simulink model "Traffic_Light_cs - 原始版本留存"  (R2020a)
settings: Solver=ode5  StartTime=0.0  StopTime=200  FixedStep=1/1000  RelTol=1e-3
PreLoadFcn:
  | mbxruntime.callbacks.PreLoadFcn(bdroot);
PostLoadFcn:
  | mbxruntime.callbacks.PostLoadFcn(bdroot);
InitFcn:
  | mbxruntime.callbacks.InitFcn(bdroot);
StartFcn:
  | mbxruntime.callbacks.StartFcn(bdroot);
StopFcn:
  | mbxruntime.callbacks.StopFcn(bdroot);
model workspace (MAT data in the model file):
  mbox_table : object (value not decoded)
  model_closed = 0
  sim_status = 0
values from neighbouring files (symbols this model uses):
  q_pass = [0 0 0 37.0489514481 49.8894252687 51.0913174965 61.791576133 65.4762304223 75.669686677 80.4628164105 88.6197377629 94.2384891559 ... (437675 elements, 87535x5)]    [Data_ckx.mat]
  q_stop = [0 0 0 15.0544571491 15.7911831418 16.0935138936 18.6666396431 19.4721381181 21.7098800606 22.5642135149 25.0883481215 26.1253405703 ... (437675 elements, 87535x5)]    [Data_ckx.mat]
  s = roadinf.s    [Constraint_T_V.m]    (also in Light_Distinguish_old.m = 75:-0.7:75-84*0.7)
undefined symbols (not defined in the file or in its folder): InitImageOutputDir, mbxruntime, sigbuilder_block, tabledata
libraries: simulink x10, PreScanSimulinkLibrary x8, simulink_extras x4, autolibshared x1, fuzblock x1
(part 3 of 5)

== system Traffic_Light_cs - 原始版本留存/CAR_Main/V2V_Input ==
  TrafficLight_ID_Main : Inport
  Light_Information1 : Inport  Tag=inport/SelfPort  Port=2  PortDimensions=3  SampleTime=1/20  BusOutputAsStruct=on
  Bus Selector1 : BusSelector  OutputSignals=ID_Ahead,LightState_Ahead,TrafficTime_Ahead
  Chart1 : Stateflow chart  TreatAsAtomicUnit=on
  Chart2 : Stateflow chart  Priority=2  TreatAsAtomicUnit=on
  MATLAB Function : MATLAB Function  Priority=1  TreatAsAtomicUnit=on
  Memory : Memory
  Memory1 : Memory
  Memory2 : Memory
  Traffic_State : Outport  VectorParamsAs1DForOutWhenUnconnected=off
  Traffic_Time : Outport  Port=2  VectorParamsAs1DForOutWhenUnconnected=off
  wires:
  Chart1/2(time) -> Traffic_Time/1
  [now_time] -> Chart1/3(now_time)
  MATLAB Function/2(Traffic_now_Time) -> [now_time]  "now_time_Main"
  [State_Next] -> Memory1/1
  [next_time] -> Chart2/3(next_time)
  Chart2/3(localnextID) -> [TrafficID_Next]
  Bus Selector1/2 -> MATLAB Function/3(Light_State_Ahead)  "<LightState_Ahead>"
  TrafficLight_ID_Main/1 -> MATLAB Function/1(Traffic_ID), Chart1/1(TrafficID), Chart2/1(TrafficID)
  [Time_Next] -> Memory2/1
  [now_state] -> Chart1/2(now_state)
  Chart2/1(state) -> [State_Next]
  Bus Selector1/1 -> MATLAB Function/2(TrafficLight_ID_Ahead)  "<ID_Ahead>"
  MATLAB Function/1(Traffic_now_State) -> [now_state]  "now_state_Main"
  MATLAB Function/4(Traffic_next_Time) -> [next_time]  "next_time_Main"
  Bus Selector1/3 -> MATLAB Function/4(Traffic_Time1)  "<TrafficTime_Ahead>"
  Chart1/1(state) -> Traffic_State/1
  Memory2/1 -> MATLAB Function/7(Time_Next)
  Memory/1 -> MATLAB Function/5(TrafficID_Next)
  Memory1/1 -> MATLAB Function/6(State_Next)
  [TrafficID_Next] -> Memory/1
  [next_state] -> Chart2/2(next_state)
  Chart2/2(time) -> [Time_Next]
  MATLAB Function/3(Traffic_next_State) -> [next_state]  "next_state_Main"
  Light_Information1/1 -> Bus Selector1/1

== system Traffic_Light_cs - 原始版本留存/CAR_Main/V2V_Output ==
  Traffic_State : Inport
  Dis_Car2Light_Main : Inport  Port=2
  Light_State_Main : Inport  Port=3
  TrafficLight_ID_Main : Inport  Port=4
  Traffic_Time : Inport  Port=5
  TrafficLight_PhaseTime : Inport  Port=6
  Bus Creator : BusCreator  Inputs=3
  Switch : Switch  Criteria=u2 > Threshold
  Switch1 : Switch  Criteria=u2 > Threshold  Threshold=500
  Traffic_Information : Outport  VectorParamsAs1DForOutWhenUnconnected=off
  "Traffic_Time " : Outport  Port=2  VectorParamsAs1DForOutWhenUnconnected=off
  wires:
  Light_State_Main/1 -> Switch1/3
  Bus Creator/1 -> Traffic_Information/1
  Traffic_State/1 -> Switch1/1
  TrafficLight_PhaseTime/1 -> Switch/3
  Switch1/1 -> Bus Creator/1  "LightState_Main"
  TrafficLight_ID_Main/1 -> Bus Creator/2  "ID_Main"
  Traffic_Time/1 -> Switch/1, Switch/2
  Dis_Car2Light_Main/1 -> Switch1/2
  Switch/1 -> Bus Creator/3, "Traffic_Time "/1  "TrafficTime_Main"

== system Traffic_Light_cs - 原始版本留存/ID_1/VISUCasingLights_Mux ==
  Green [-] : Inport  Tag=inport/Green [-]  SampleTime=1/1000  BusOutputAsStruct=on
  Orange [-] : Inport  Tag=inport/Orange [-]  Port=2  SampleTime=1/1000  BusOutputAsStruct=on
  Red [-] : Inport  Tag=inport/Red [-]  Port=3  SampleTime=1/1000  BusOutputAsStruct=on
  MuxVisuLights : Mux  Inputs=3
  VISUCasingLights_ID_1 : Outport  Tag=outport/VisuCasingLights  SampleTime=1/1000
  wires:
  MuxVisuLights/1 -> VISUCasingLights_ID_1/1
  Green [-]/1 -> MuxVisuLights/1
  Orange [-]/1 -> MuxVisuLights/2
  Red [-]/1 -> MuxVisuLights/3

== system Traffic_Light_cs - 原始版本留存/ID_2/VISUCasingLights_Mux ==
  Green [-] : Inport  Tag=inport/Green [-]  SampleTime=1/1000  BusOutputAsStruct=on
  Orange [-] : Inport  Tag=inport/Orange [-]  Port=2  SampleTime=1/1000  BusOutputAsStruct=on
  Red [-] : Inport  Tag=inport/Red [-]  Port=3  SampleTime=1/1000  BusOutputAsStruct=on
  MuxVisuLights : Mux  Inputs=3
  VISUCasingLights_ID_2 : Outport  Tag=outport/VisuCasingLights  SampleTime=1/1000
  wires:
  MuxVisuLights/1 -> VISUCasingLights_ID_2/1
  Green [-]/1 -> MuxVisuLights/1
  Orange [-]/1 -> MuxVisuLights/2
  Red [-]/1 -> MuxVisuLights/3

== system Traffic_Light_cs - 原始版本留存/ID_3/VISUCasingLights_Mux ==
  Green [-] : Inport  Tag=inport/Green [-]  SampleTime=1/1000  BusOutputAsStruct=on
  Orange [-] : Inport  Tag=inport/Orange [-]  Port=2  SampleTime=1/1000  BusOutputAsStruct=on
  Red [-] : Inport  Tag=inport/Red [-]  Port=3  SampleTime=1/1000  BusOutputAsStruct=on
  MuxVisuLights : Mux  Inputs=3
  VISUCasingLights_ID_3 : Outport  Tag=outport/VisuCasingLights  SampleTime=1/1000
  wires:
  MuxVisuLights/1 -> VISUCasingLights_ID_3/1
  Green [-]/1 -> MuxVisuLights/1
  Orange [-]/1 -> MuxVisuLights/2
  Red [-]/1 -> MuxVisuLights/3

== system Traffic_Light_cs - 原始版本留存/VISUCasingLights_ID_1/Actuator ==
  VISUCasingLights_ID_1 : Inport  Tag=inport/VisuCasingLights  SampleTime=1/1000  BusOutputAsStruct=on
  DemuxVisuLights : Demux  Outputs=3
  LimiterVisuLights : Saturate  UpperLimit=1  LowerLimit=0
  visu_Green [-] : S-Function  FunctionName=sfun_MaterialColorSelector  Parameters=mbxruntime.parameters.convert(UniqueID), mbxruntime.parameters.convert(ColorsObjectQuery), mbxruntime.parameters.convert(Colors),tabledata, TimeStep  SFunctionDeploymentMode=off  EnableBusSupport=off  mask(PreScan Sink Block: VisuTrafficLight){UniqueID=35, ColorsObjectQuery=child:name=ID_1.Casing.LightGreen, Colors=[5   32   25  255    0   64   50  255    0   64   50  255    0    0    0  255; 0   45   34  255    0   45   34  255    0   45   34  255   30  306  240  255], TimeStep=1/1000}
      mask prompts: UniqueID "Parent Unique Identifier"; ColorsObjectQuery "Query for Color Object"; Colors "Matrix of colors"; TimeStep "Simulink time step"
      mask help:
      | The VisuTrafficLight block provides a way to animate traffic lights: switch on and off individual lights.
      |
      | For more information, please click Help.
      mask init:
      | [tabledata] = mbxruntime.parameters.table(UniqueID,ColorsObjectQuery,Colors);
      mask Help: eval('openHelp(731)')
      mask Display: image(imread('TrafficLightCasing.png'))
  visu_Orange [-] : S-Function  FunctionName=sfun_MaterialColorSelector  Parameters=mbxruntime.parameters.convert(UniqueID), mbxruntime.parameters.convert(ColorsObjectQuery), mbxruntime.parameters.convert(Colors),tabledata, TimeStep  SFunctionDeploymentMode=off  EnableBusSupport=off  mask(PreScan Sink Block: VisuTrafficLight){UniqueID=35, ColorsObjectQuery=child:name=ID_1.Casing.LightOrange, Colors=[32   25    5  255   64   48    5  255   64   54    5  255    0    0    0  255; 45   34    0  255   45   34    0  255   45   34    0  255  306  229    5  255], TimeStep=1/1000}
      mask prompts: UniqueID "Parent Unique Identifier"; ColorsObjectQuery "Query for Color Object"; Colors "Matrix of colors"; TimeStep "Simulink time step"
      mask help:
      | The VisuTrafficLight block provides a way to animate traffic lights: switch on and off individual lights.
      |
      | For more information, please click Help.
      mask init:
      | [tabledata] = mbxruntime.parameters.table(UniqueID,ColorsObjectQuery,Colors);
      mask Help: eval('openHelp(731)')
      mask Display: image(imread('TrafficLightCasing.png'))
  visu_Red [-] : S-Function  FunctionName=sfun_MaterialColorSelector  Parameters=mbxruntime.parameters.convert(UniqueID), mbxruntime.parameters.convert(ColorsObjectQuery), mbxruntime.parameters.convert(Colors),tabledata, TimeStep  SFunctionDeploymentMode=off  EnableBusSupport=off  mask(PreScan Sink Block: VisuTrafficLight){UniqueID=35, ColorsObjectQuery=child:name=ID_1.Casing.LightRed, Colors=[32    5    5  255   64    5    5  255   64    5    5  255    0    0    0  255; 45    0    0  255   45    0    0  255   45    0    0  255  306   30   30  255], TimeStep=1/1000}
      mask prompts: UniqueID "Parent Unique Identifier"; ColorsObjectQuery "Query for Color Object"; Colors "Matrix of colors"; TimeStep "Simulink time step"
      mask help:
      | The VisuTrafficLight block provides a way to animate traffic lights: switch on and off individual lights.
      |
      | For more information, please click Help.
      mask init:
      | [tabledata] = mbxruntime.parameters.table(UniqueID,ColorsObjectQuery,Colors);
      mask Help: eval('openHelp(731)')
      mask Display: image(imread('TrafficLightCasing.png'))
  wires:
  VISUCasingLights_ID_1/1 -> LimiterVisuLights/1
  LimiterVisuLights/1 -> DemuxVisuLights/1
  DemuxVisuLights/1 -> visu_Green [-]/1
  DemuxVisuLights/2 -> visu_Orange [-]/1
  DemuxVisuLights/3 -> visu_Red [-]/1

== system Traffic_Light_cs - 原始版本留存/VISUCasingLights_ID_2/Actuator ==
  VISUCasingLights_ID_2 : Inport  Tag=inport/VisuCasingLights  SampleTime=1/1000  BusOutputAsStruct=on
  DemuxVisuLights : Demux  Outputs=3
  LimiterVisuLights : Saturate  UpperLimit=1  LowerLimit=0
  visu_Green [-] : S-Function  FunctionName=sfun_MaterialColorSelector  Parameters=mbxruntime.parameters.convert(UniqueID), mbxruntime.parameters.convert(ColorsObjectQuery), mbxruntime.parameters.convert(Colors),tabledata, TimeStep  SFunctionDeploymentMode=off  EnableBusSupport=off  mask(PreScan Sink Block: VisuTrafficLight){UniqueID=525, ColorsObjectQuery=child:name=ID_2.Casing.LightGreen, Colors=[5   32   25  255    0   64   50  255    0   64   50  255    0    0    0  255; 0   45   34  255    0   45   34  255    0   45   34  255   30  306  240  255], TimeStep=1/1000}
      mask prompts: UniqueID "Parent Unique Identifier"; ColorsObjectQuery "Query for Color Object"; Colors "Matrix of colors"; TimeStep "Simulink time step"
      mask help:
      | The VisuTrafficLight block provides a way to animate traffic lights: switch on and off individual lights.
      |
      | For more information, please click Help.
      mask init:
      | [tabledata] = mbxruntime.parameters.table(UniqueID,ColorsObjectQuery,Colors);
      mask Help: eval('openHelp(731)')
      mask Display: image(imread('TrafficLightCasing.png'))
  visu_Orange [-] : S-Function  FunctionName=sfun_MaterialColorSelector  Parameters=mbxruntime.parameters.convert(UniqueID), mbxruntime.parameters.convert(ColorsObjectQuery), mbxruntime.parameters.convert(Colors),tabledata, TimeStep  SFunctionDeploymentMode=off  EnableBusSupport=off  mask(PreScan Sink Block: VisuTrafficLight){UniqueID=525, ColorsObjectQuery=child:name=ID_2.Casing.LightOrange, Colors=[32   25    5  255   64   48    5  255   64   54    5  255    0    0    0  255; 45   34    0  255   45   34    0  255   45   34    0  255  306  229    5  255], TimeStep=1/1000}
      mask prompts: UniqueID "Parent Unique Identifier"; ColorsObjectQuery "Query for Color Object"; Colors "Matrix of colors"; TimeStep "Simulink time step"
      mask help:
      | The VisuTrafficLight block provides a way to animate traffic lights: switch on and off individual lights.
      |
      | For more information, please click Help.
      mask init:
      | [tabledata] = mbxruntime.parameters.table(UniqueID,ColorsObjectQuery,Colors);
      mask Help: eval('openHelp(731)')
      mask Display: image(imread('TrafficLightCasing.png'))
  visu_Red [-] : S-Function  FunctionName=sfun_MaterialColorSelector  Parameters=mbxruntime.parameters.convert(UniqueID), mbxruntime.parameters.convert(ColorsObjectQuery), mbxruntime.parameters.convert(Colors),tabledata, TimeStep  SFunctionDeploymentMode=off  EnableBusSupport=off  mask(PreScan Sink Block: VisuTrafficLight){UniqueID=525, ColorsObjectQuery=child:name=ID_2.Casing.LightRed, Colors=[32    5    5  255   64    5    5  255   64    5    5  255    0    0    0  255; 45    0    0  255   45    0    0  255   45    0    0  255  306   30   30  255], TimeStep=1/1000}
      mask prompts: UniqueID "Parent Unique Identifier"; ColorsObjectQuery "Query for Color Object"; Colors "Matrix of colors"; TimeStep "Simulink time step"
      mask help:
      | The VisuTrafficLight block provides a way to animate traffic lights: switch on and off individual lights.
      |
      | For more information, please click Help.
      mask init:
      | [tabledata] = mbxruntime.parameters.table(UniqueID,ColorsObjectQuery,Colors);
      mask Help: eval('openHelp(731)')
      mask Display: image(imread('TrafficLightCasing.png'))
  wires:
  VISUCasingLights_ID_2/1 -> LimiterVisuLights/1
  LimiterVisuLights/1 -> DemuxVisuLights/1
  DemuxVisuLights/1 -> visu_Green [-]/1
  DemuxVisuLights/2 -> visu_Orange [-]/1
  DemuxVisuLights/3 -> visu_Red [-]/1

== system Traffic_Light_cs - 原始版本留存/VISUCasingLights_ID_3/Actuator ==
  VISUCasingLights_ID_3 : Inport  Tag=inport/VisuCasingLights  SampleTime=1/1000  BusOutputAsStruct=on
  DemuxVisuLights : Demux  Outputs=3
  LimiterVisuLights : Saturate  UpperLimit=1  LowerLimit=0
  visu_Green [-] : S-Function  FunctionName=sfun_MaterialColorSelector  Parameters=mbxruntime.parameters.convert(UniqueID), mbxruntime.parameters.convert(ColorsObjectQuery), mbxruntime.parameters.convert(Colors),tabledata, TimeStep  SFunctionDeploymentMode=off  EnableBusSupport=off  mask(PreScan Sink Block: VisuTrafficLight){UniqueID=526, ColorsObjectQuery=child:name=ID_3.Casing.LightGreen, Colors=[5   32   25  255    0   64   50  255    0   64   50  255    0    0    0  255; 0   45   34  255    0   45   34  255    0   45   34  255   30  306  240  255], TimeStep=1/1000}
      mask prompts: UniqueID "Parent Unique Identifier"; ColorsObjectQuery "Query for Color Object"; Colors "Matrix of colors"; TimeStep "Simulink time step"
      mask help:
      | The VisuTrafficLight block provides a way to animate traffic lights: switch on and off individual lights.
      |
      | For more information, please click Help.
      mask init:
      | [tabledata] = mbxruntime.parameters.table(UniqueID,ColorsObjectQuery,Colors);
      mask Help: eval('openHelp(731)')
      mask Display: image(imread('TrafficLightCasing.png'))
  visu_Orange [-] : S-Function  FunctionName=sfun_MaterialColorSelector  Parameters=mbxruntime.parameters.convert(UniqueID), mbxruntime.parameters.convert(ColorsObjectQuery), mbxruntime.parameters.convert(Colors),tabledata, TimeStep  SFunctionDeploymentMode=off  EnableBusSupport=off  mask(PreScan Sink Block: VisuTrafficLight){UniqueID=526, ColorsObjectQuery=child:name=ID_3.Casing.LightOrange, Colors=[32   25    5  255   64   48    5  255   64   54    5  255    0    0    0  255; 45   34    0  255   45   34    0  255   45   34    0  255  306  229    5  255], TimeStep=1/1000}
      mask prompts: UniqueID "Parent Unique Identifier"; ColorsObjectQuery "Query for Color Object"; Colors "Matrix of colors"; TimeStep "Simulink time step"
      mask help:
      | The VisuTrafficLight block provides a way to animate traffic lights: switch on and off individual lights.
      |
      | For more information, please click Help.
      mask init:
      | [tabledata] = mbxruntime.parameters.table(UniqueID,ColorsObjectQuery,Colors);
      mask Help: eval('openHelp(731)')
      mask Display: image(imread('TrafficLightCasing.png'))
  visu_Red [-] : S-Function  FunctionName=sfun_MaterialColorSelector  Parameters=mbxruntime.parameters.convert(UniqueID), mbxruntime.parameters.convert(ColorsObjectQuery), mbxruntime.parameters.convert(Colors),tabledata, TimeStep  SFunctionDeploymentMode=off  EnableBusSupport=off  mask(PreScan Sink Block: VisuTrafficLight){UniqueID=526, ColorsObjectQuery=child:name=ID_3.Casing.LightRed, Colors=[32    5    5  255   64    5    5  255   64    5    5  255    0    0    0  255; 45    0    0  255   45    0    0  255   45    0    0  255  306   30   30  255], TimeStep=1/1000}
      mask prompts: UniqueID "Parent Unique Identifier"; ColorsObjectQuery "Query for Color Object"; Colors "Matrix of colors"; TimeStep "Simulink time step"
      mask help:
      | The VisuTrafficLight block provides a way to animate traffic lights: switch on and off individual lights.
      |
      | For more information, please click Help.
      mask init:
      | [tabledata] = mbxruntime.parameters.table(UniqueID,ColorsObjectQuery,Colors);
      mask Help: eval('openHelp(731)')
      mask Display: image(imread('TrafficLightCasing.png'))
  wires:
  VISUCasingLights_ID_3/1 -> LimiterVisuLights/1
  LimiterVisuLights/1 -> DemuxVisuLights/1
  DemuxVisuLights/1 -> visu_Green [-]/1
  DemuxVisuLights/2 -> visu_Orange [-]/1
  DemuxVisuLights/3 -> visu_Red [-]/1

== system Traffic_Light_cs - 原始版本留存/CAR_Ahead/Decision/Function-Call Subsystem ==
  Dis : Inport
  "CameraSensor " : Inport  Port=2
  Traffic_State : Inport  Port=3
  Traffic_Time : Inport  Port=4
  V_now : Inport  Port=5
  function : TriggerPort  TriggerType=function-call  VariantControl=Variant
  Chart : Stateflow chart  TreatAsAtomicUnit=on
  Subsystem : Subsystem
  Switch : Switch  Criteria=u2 > Threshold
  Terminator : Terminator
  Terminator1 : Terminator
  Light_State_Ahead : Outport  VectorParamsAs1DForOutWhenUnconnected=off
  wires:
  V_now/1 -> Terminator1/1
  Traffic_Time/1 -> Terminator/1, [TrafficTime]
  Subsystem/1(Light_State_Ahead) -> Switch/3
  Switch/1 -> Light_State_Ahead/1, [LightState]
  Chart/1(Camera_Call()) -> Subsystem/Trigger
  Traffic_State/1 -> Chart/1(Traffic_State), Switch/1, Switch/2
  "CameraSensor "/1 -> Subsystem/2("CameraSensor ")
  Dis/1 -> Subsystem/1(Dis), [Distance]

== system Traffic_Light_cs - 原始版本留存/CAR_Ahead/SELF_Demux/compas converter ==
  rotz [rad] : Inport
  cart2compas : Subsystem
  rad2deg : Gain  Gain=180/pi
  heading [deg] : Outport
  wires:
  rad2deg/1 -> cart2compas/1(Angle [deg])
  rotz [rad]/1 -> rad2deg/1
  cart2compas/1(heading [deg]) -> heading [deg]/1

== system Traffic_Light_cs - 原始版本留存/CAR_Ahead/Subsystem/Signal Builder ==
  Demux : Demux  Tag=STV Demux  Outputs=6
      settings: DisplayOption=none
  FromWs : FromWorkspace  Tag=STV FromWs  VariableName=tuvar
      SigBuilderData=|
      | common.afterFinalStr = 'Extrapolate'
      | common.sampleTime = 0
      | dataSet.timeRange = [0 200]
      | dataSet.name = 'Traffic Light GPS Information'
      | sbobj.Groups.Name = 'Traffic Light GPS Information'
      | sbobj.Groups.Signals(1).Name = 'ID==1,X'
      | sbobj.Groups.Signals(1).XData = [0 200]
      | sbobj.Groups.Signals(1).YData = [-610.5 -610.5]
      | sbobj.Groups.Signals(2).Name = 'ID==1,Y'
      | sbobj.Groups.Signals(2).XData = [0 200]
      | sbobj.Groups.Signals(2).YData = [362.27 362.27]
      | sbobj.Groups.Signals(3).Name = 'ID==2,X'
      | sbobj.Groups.Signals(3).XData = [0 200]
      | sbobj.Groups.Signals(3).YData = [-639.42 -639.42]
      | sbobj.Groups.Signals(4).Name = 'ID==2,Y'
      | sbobj.Groups.Signals(4).XData = [0 200]
      | sbobj.Groups.Signals(4).YData = [295.94 295.94]
      | sbobj.Groups.Signals(5).Name = 'ID==3,X'
      | sbobj.Groups.Signals(5).XData = [0 200]
      | sbobj.Groups.Signals(5).YData = [-718.98 -718.98]
      | sbobj.Groups.Signals(6).Name = 'ID==3,Y'
      | sbobj.Groups.Signals(6).XData = [0 200]
      | sbobj.Groups.Signals(6).YData = [201.74 201.74]
      | sbobj.Groups.TimeRange = [0 200]
  ID==1,X : Outport  Tag=STV Outport
  ID==1,Y : Outport  Tag=STV Outport  Port=2  VectorParamsAs1DForOutWhenUnconnected=off
  ID==2,X : Outport  Tag=STV Outport  Port=3  VectorParamsAs1DForOutWhenUnconnected=off
  ID==2,Y : Outport  Tag=STV Outport  Port=4  VectorParamsAs1DForOutWhenUnconnected=off
  ID==3,X : Outport  Tag=STV Outport  Port=5  VectorParamsAs1DForOutWhenUnconnected=off
  ID==3,Y : Outport  Tag=STV Outport  Port=6  VectorParamsAs1DForOutWhenUnconnected=off
  wires:
  Demux/6 -> ID==3,Y/1
  Demux/5 -> ID==3,X/1
  Demux/4 -> ID==2,Y/1
  Demux/3 -> ID==2,X/1
  Demux/2 -> ID==1,Y/1
  Demux/1 -> ID==1,X/1
  FromWs/1 -> Demux/1

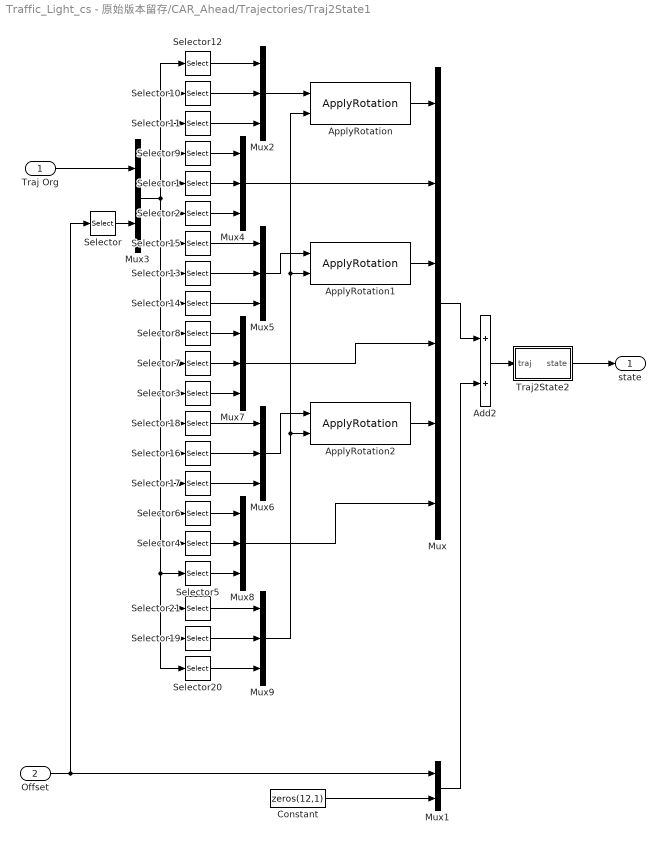
== system Traffic_Light_cs - 原始版本留存/CAR_Ahead/Trajectories/Traj2State1 ==
  Traj Org : Inport
  Offset : Inport  Port=2
  Add2 : Sum
  ApplyRotation : PreScanSimulinkLibrary/ApplyRotation  SystemSampleTime=-1  Latency=0  AutoFrameSizeCalculation=off
  ApplyRotation1 : PreScanSimulinkLibrary/ApplyRotation  SystemSampleTime=-1  Latency=0  AutoFrameSizeCalculation=off
  ApplyRotation2 : PreScanSimulinkLibrary/ApplyRotation  SystemSampleTime=-1  Latency=0  AutoFrameSizeCalculation=off
  Constant : Constant  Value=zeros(12,1)
  Mux : Mux  Inputs=6
  Mux1 : Mux  Inputs=2
  Mux{2,4..9} (7 alike) : Mux  Inputs=3
  Mux3 : Mux  Inputs=2
  Selector : Selector  InputPortWidth=6  IndexOptions=Index vector (dialog)  Indices=[4 5 6]  OutputSizes=1
  Selector1 : Selector  InputPortWidth=21  IndexOptions=Index vector (dialog)  Indices=[5]  OutputSizes=1
  Selector10 : Selector  InputPortWidth=21  IndexOptions=Index vector (dialog)  Indices=[2]  OutputSizes=1
  Selector11 : Selector  InputPortWidth=21  IndexOptions=Index vector (dialog)  Indices=[3]  OutputSizes=1
  Selector12 : Selector  InputPortWidth=21  IndexOptions=Index vector (dialog)  Indices=[1]  OutputSizes=1
  Selector13 : Selector  InputPortWidth=21  IndexOptions=Index vector (dialog)  Indices=[8]  OutputSizes=1
  Selector14 : Selector  InputPortWidth=21  IndexOptions=Index vector (dialog)  Indices=[9]  OutputSizes=1
  Selector15 : Selector  InputPortWidth=21  IndexOptions=Index vector (dialog)  Indices=[7]  OutputSizes=1
  Selector16 : Selector  InputPortWidth=21  IndexOptions=Index vector (dialog)  Indices=[14]  OutputSizes=1
  Selector17 : Selector  InputPortWidth=21  IndexOptions=Index vector (dialog)  Indices=[15]  OutputSizes=1
  Selector18 : Selector  InputPortWidth=21  IndexOptions=Index vector (dialog)  Indices=[13]  OutputSizes=1
  Selector19 : Selector  InputPortWidth=21  IndexOptions=Index vector (dialog)  Indices=[20]  OutputSizes=1
  Selector2 : Selector  InputPortWidth=21  IndexOptions=Index vector (dialog)  Indices=[6]  OutputSizes=1
  Selector20 : Selector  InputPortWidth=21  IndexOptions=Index vector (dialog)  Indices=[21]  OutputSizes=1
  Selector21 : Selector  InputPortWidth=21  IndexOptions=Index vector (dialog)  Indices=[19]  OutputSizes=1
  Selector3 : Selector  InputPortWidth=21  IndexOptions=Index vector (dialog)  Indices=[12]  OutputSizes=1
  Selector4 : Selector  InputPortWidth=21  IndexOptions=Index vector (dialog)  Indices=[17]  OutputSizes=1
  Selector5 : Selector  InputPortWidth=21  IndexOptions=Index vector (dialog)  Indices=[18]  OutputSizes=1
  Selector6 : Selector  InputPortWidth=21  IndexOptions=Index vector (dialog)  Indices=[16]  OutputSizes=1
  Selector7 : Selector  InputPortWidth=21  IndexOptions=Index vector (dialog)  Indices=[11]  OutputSizes=1
  Selector8 : Selector  InputPortWidth=21  IndexOptions=Index vector (dialog)  Indices=[10]  OutputSizes=1
  Selector9 : Selector  InputPortWidth=21  IndexOptions=Index vector (dialog)  Indices=[4]  OutputSizes=1
  Traj2State2 : Subsystem
  state : Outport
  wires:
  Mux9/1 -> ApplyRotation2/2, ApplyRotation1/2, ApplyRotation/2
  Selector20/1 -> Mux9/3
  Selector19/1 -> Mux9/2
  Selector21/1 -> Mux9/1
  Selector5/1 -> Mux8/3
  Selector4/1 -> Mux8/2
  Selector6/1 -> Mux8/1
  Mux8/1 -> Mux/6
  Mux6/1 -> ApplyRotation2/1
  Mux7/1 -> Mux/4
  ApplyRotation2/1 -> Mux/5
  Selector3/1 -> Mux7/3
  Selector7/1 -> Mux7/2
  Selector8/1 -> Mux7/1
  Mux4/1 -> Mux/2
  Mux5/1 -> ApplyRotation1/1
  ApplyRotation1/1 -> Mux/3
  Mux2/1 -> ApplyRotation/1
  ApplyRotation/1 -> Mux/1
  Selector2/1 -> Mux4/3
  Selector1/1 -> Mux4/2
  Selector9/1 -> Mux4/1
  Selector17/1 -> Mux6/3
  Selector16/1 -> Mux6/2
  Selector18/1 -> Mux6/1
  Selector14/1 -> Mux5/3
  Selector13/1 -> Mux5/2
  Selector15/1 -> Mux5/1
  Selector11/1 -> Mux2/3
  Selector10/1 -> Mux2/2
  Selector12/1 -> Mux2/1
  Mux3/1 -> Selector8/1, Selector7/1, Selector3/1, Selector18/1, Selector16/1, Selector17/1, Selector6/1, Selector20/1, Selector19/1, Selector21/1, Selector5/1, Selector4/1, Selector14/1, Selector13/1, Selector15/1, Selector2/1, Selector1/1, Selector9/1, Selector12/1, Selector10/1, Selector11/1
  Mux1/1 -> Add2/2
  Constant/1 -> Mux1/2
  Add2/1 -> Traj2State2/1(traj)
  Selector/1 -> Mux3/2
  Traj Org/1 -> Mux3/1
  Offset/1 -> Mux1/1, Selector/1
  Mux/1 -> Add2/1
  Traj2State2/1(state) -> state/1

== system Traffic_Light_cs - 原始版本留存/CAR_Ahead/Trajectories/TrajCoGOffset ==
  State In : Inport
  Add : Sum  Inputs=+-+
  Add1 : Sum
  ApplyRotation : PreScanSimulinkLibrary/ApplyRotation  SystemSampleTime=-1  Latency=0  AutoFrameSizeCalculation=off
  ApplyRotation1 : PreScanSimulinkLibrary/ApplyRotation  SystemSampleTime=-1  Latency=0  AutoFrameSizeCalculation=off
  CoG Offset : Constant  Value=[0 0 CoGOffsetZ]
  Degrees to Radians : simulink_extras/Transformations/Degrees to Radians
  Demux1 : Demux  Outputs=[3 3 3]
  Mux : Mux  Inputs=[3 3 3]
  Orientation : Constant  Value=[InitRoll InitPitch 0]
  State Out : Outport
  wires:
  State In/1 -> Demux1/1
  Demux1/1 -> Add/1
  Add/1 -> Mux/1
  Demux1/3 -> Mux/3, Add1/2
  Mux/1 -> State Out/1
  Demux1/2 -> Mux/2
  Orientation/1 -> Degrees to Radians/1
  ApplyRotation/1 -> Add/3
  ApplyRotation1/1 -> Add/2
  Add1/1 -> ApplyRotation/2
  CoG Offset/1 -> ApplyRotation1/1, ApplyRotation/1
  Degrees to Radians/1 -> Add1/1, ApplyRotation1/2

== system Traffic_Light_cs - 原始版本留存/CAR_Ahead/Trajectories/Trajectory_1 ==
  From Workspace : FromWorkspace  VariableName=trajectory  SampleTime=TimeStep  ZeroCross=off  OutputAfterFinalValue=Holding final value
  From Workspace1 : FromWorkspace  VariableName=trajectory  SampleTime=TimeStep  ZeroCross=off  OutputAfterFinalValue=Setting to zero
  Mux : Mux  Inputs=2
  Selector1 : Selector  InputPortWidth=24  IndexOptions=Index vector (dialog)  Indices=[7:18]  OutputSizes=1
  Selector9 : Selector  InputPortWidth=24  IndexOptions=Index vector (dialog)  Indices=[1:6]  OutputSizes=1
  trajectory : Outport
  wires:
  From Workspace/1 -> Selector9/1
  From Workspace1/1 -> Selector1/1
  Mux/1 -> trajectory/1
  Selector9/1 -> Mux/1
  Selector1/1 -> Mux/2

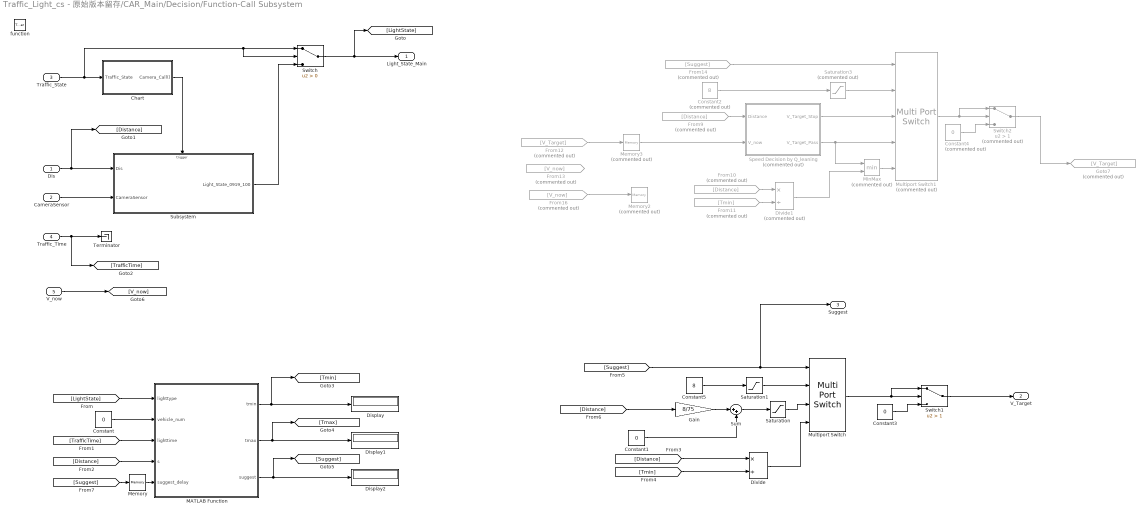
== system Traffic_Light_cs - 原始版本留存/CAR_Main/Decision/Function-Call Subsystem ==
  Dis : Inport
  "CameraSensor " : Inport  Port=2
  Traffic_State : Inport  Port=3
  Traffic_Time : Inport  Port=4
  V_now : Inport  Port=5
  function : TriggerPort  TriggerType=function-call  VariantControl=Variant
  Chart : Stateflow chart  TreatAsAtomicUnit=on
  Constant : Constant  Value=0
  Constant1 : Constant  Value=0
  Constant2 : Constant  Commented=on  Value=8
  Constant3 : Constant  Value=0
  Constant4 : Constant  Commented=on  Value=0
  Constant5 : Constant  Value=8
  Display : Display
  Display1 : Display
  Display2 : Display
  Divide : Product  Inputs=*/
  Divide1 : Product  Commented=on  Inputs=*/
  From10 : From  Commented=on  GotoTag=Distance
  From11 : From  Commented=on  GotoTag=Tmin
  From12 : From  Commented=on  GotoTag=V_Target
  From13 : From  Commented=on  GotoTag=V_now
  From14 : From  Commented=on  GotoTag=Suggest
  From16 : From  Commented=on  GotoTag=V_now
  From9 : From  Commented=on  GotoTag=Distance
  Gain : Gain  Gain=8/75
  Goto7 : Goto  Commented=on  GotoTag=V_Target
  MATLAB Function : MATLAB Function  TreatAsAtomicUnit=on
  Memory : Memory  InheritSampleTime=on
  Memory2 : Memory  Commented=on  InitialCondition=6  InheritSampleTime=on
  Memory3 : Memory  Commented=on  InitialCondition=3  InheritSampleTime=on
  MinMax : MinMax  Commented=on  Inputs=2
  Multiport Switch : MultiPortSwitch  DataPortOrder=Specify indices  DataPortIndices={-1,4,3}  DiagnosticForDefault=None
  Multiport Switch1 : MultiPortSwitch  Commented=on  DataPortOrder=Specify indices  DataPortIndices={-1,4,1,3}  DiagnosticForDefault=None
  Saturation : Saturate  UpperLimit=10  LowerLimit=0
  Saturation1 : Saturate  UpperLimit=20  LowerLimit=5
  Saturation3 : Saturate  Commented=on  UpperLimit=20  LowerLimit=0
  Speed Decision by Q_leaning : Subsystem  Commented=on
  Subsystem : Subsystem
  Sum : Sum  Inputs=|++
  Switch : Switch  Criteria=u2 > Threshold
  Switch1 : Switch  Criteria=u2 > Threshold  Threshold=1
  Switch2 : Switch  Commented=on  Criteria=u2 > Threshold  Threshold=1
  Terminator : Terminator
  Light_State_Main : Outport  VectorParamsAs1DForOutWhenUnconnected=off
  V_Target : Outport  Port=2  VectorParamsAs1DForOutWhenUnconnected=off
  "Suggest " : Outport  Port=3  VectorParamsAs1DForOutWhenUnconnected=off
  wires:
  Constant5/1 -> Saturation1/1
  Switch1/1 -> V_Target/1
  Constant2/1 -> Saturation3/1
  Memory3/1 -> Speed Decision by Q_leaning/2(V_now)
  From12/1 -> Memory3/1
  From16/1 -> Memory2/1
  MinMax/1 -> Multiport Switch1/5
  Divide1/1 -> MinMax/2
  Speed Decision by Q_leaning/2(V_Target_Pass) -> Multiport Switch1/4, MinMax/1
  From10/1 -> Divide1/1
  From11/1 -> Divide1/2
  V_now/1 -> [V_now]
  Speed Decision by Q_leaning/1(V_Target_Stop) -> Multiport Switch1/3
  From9/1 -> Speed Decision by Q_leaning/1(Distance)
  From14/1 -> Multiport Switch1/1
  Multiport Switch1/1 -> Switch2/2, Switch2/1
  Constant4/1 -> Switch2/3
  Saturation3/1 -> Multiport Switch1/2
  Switch2/1 -> Goto7/1
  Saturation1/1 -> Multiport Switch/2
  Constant3/1 -> Switch1/3
  Multiport Switch/1 -> Switch1/2, Switch1/1
  Memory/1 -> MATLAB Function/5(suggest_delay)
  [Suggest] -> Memory/1
  Sum/1 -> Saturation/1
  Gain/1 -> Sum/1
  [Distance] -> Gain/1
  Constant1/1 -> Sum/2
  Saturation/1 -> Multiport Switch/3
  [Suggest] -> Multiport Switch/1, "Suggest "/1
  Divide/1 -> Multiport Switch/4
  [Tmin] -> Divide/2
  [Distance] -> Divide/1
  MATLAB Function/3(suggest) -> Display2/1, [Suggest]
  MATLAB Function/2(tmax) -> Display1/1, [Tmax]
  MATLAB Function/1(tmin) -> Display/1, [Tmin]
  [Distance] -> MATLAB Function/4(s)
  Constant/1 -> MATLAB Function/2(vehicle_num)
  [TrafficTime] -> MATLAB Function/3(lighttime)
  [LightState] -> MATLAB Function/1(lighttype)
  Traffic_Time/1 -> Terminator/1, [TrafficTime]
  Subsystem/1(Light_State_0919_100) -> Switch/3
  Switch/1 -> Light_State_Main/1, [LightState]
  Chart/1(Camera_Call()) -> Subsystem/Trigger
  Traffic_State/1 -> Chart/1(Traffic_State), Switch/1, Switch/2
  "CameraSensor "/1 -> Subsystem/2("CameraSensor ")
  Dis/1 -> Subsystem/1(Dis), [Distance]

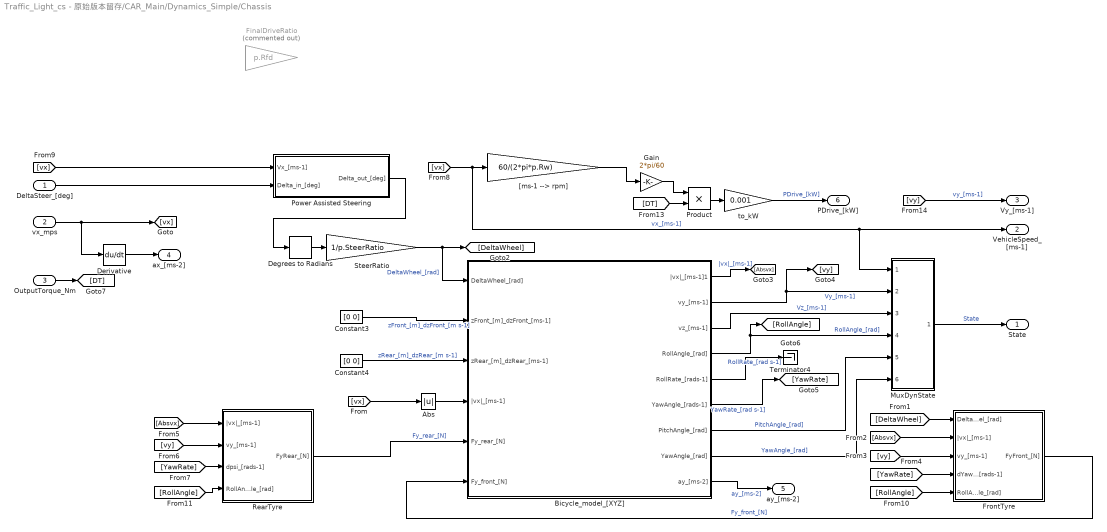
== system Traffic_Light_cs - 原始版本留存/CAR_Main/Dynamics_Simple/Chassis ==
  DeltaSteer_[deg] : Inport
  vx_mps : Inport  Port=2
  OutputTorque_Nm : Inport  Port=3
  Abs : Abs
  Bicycle_model_[XYZ] : Subsystem
      mask Display: image(imread('Bicycle_model.png'));
  Constant3 : Constant  Value=[0 0]
  Constant4 : Constant  Value=[0 0]
  Degrees to Radians : simulink_extras/Transformations/Degrees to Radians
  Derivative : Derivative
  "FinalDriveRatio " : Gain  Commented=on  Gain=p.Rfd  SaturateOnIntegerOverflow=on  OutDataTypeStr=Inherit: Same as input  ParamDataTypeStr=Inherit: Same as input
  FrontTyre : Subsystem
      mask Display: image(imread('Tyre.png'));
  Gain : Gain  Gain=2*pi/60
  MuxDynState : Subsystem
  Power Assisted Steering : Subsystem
  Product : Product  RndMeth=Zero
  RearTyre : Subsystem
      mask Display: image(imread('Tyre.png'));
  SteerRatio : Gain  Gain=1/p.SteerRatio
  Terminator4 : Terminator
  "[ms-1 --> rpm]" : Gain  Gain=60/(2*pi*p.Rw)  SaturateOnIntegerOverflow=on  OutDataTypeStr=Inherit: Same as input  ParamDataTypeStr=Inherit: Same as input
  to_kW : Gain  Gain=0.001
  State : Outport  VectorParamsAs1DForOutWhenUnconnected=off
  VehicleSpeed_[ms-1] : Outport  Port=2  VectorParamsAs1DForOutWhenUnconnected=off
  Vy_[ms-1] : Outport  Port=3  VectorParamsAs1DForOutWhenUnconnected=off
  ax_[ms-2] : Outport  Port=4  VectorParamsAs1DForOutWhenUnconnected=off
  ay_[ms-2] : Outport  Port=5  VectorParamsAs1DForOutWhenUnconnected=off
  PDrive_[kW] : Outport  Port=6  VectorParamsAs1DForOutWhenUnconnected=off
  wires:
  Derivative/1 -> ax_[ms-2]/1
  OutputTorque_Nm/1 -> [DT]
  vx_mps/1 -> [vx], Derivative/1
  MuxDynState/1(State) -> State/1  "State"
  Bicycle_model_[XYZ]/5(RollRate_[rads-1]) -> Terminator4/1  "RollRate_[rad s-1]"
  Constant4/1 -> Bicycle_model_[XYZ]/3(zRear_[m]_dzRear_[ms-1])  "zRear_[m]_dzRear_[m s-1]"
  Constant3/1 -> Bicycle_model_[XYZ]/2(zFront_[m]_dzFront_[ms-1])  "zFront_[m]_dzFront_[m s-1]"
  [RollAngle] -> RearTyre/4(RollAngle_[rad])
  [RollAngle] -> FrontTyre/5(RollAngle_[rad])
  Power Assisted Steering/1(Delta_out_[deg]) -> Degrees to Radians/1
  DeltaSteer_[deg]/1 -> Power Assisted Steering/2(Delta_in_[deg])
  [vx] -> Power Assisted Steering/1(Vx_[ms-1])
  [vx] -> MuxDynState/1(vx [ms-1]), VehicleSpeed_[ms-1]/1, "[ms-1 --> rpm]"/1  "vx_[ms-1]"
  "[ms-1 --> rpm]"/1 -> Gain/1
  Bicycle_model_[XYZ]/8(YawAngle_[rad]) -> MuxDynState/6(Y [rad])  "YawAngle_[rad]"
  Bicycle_model_[XYZ]/7(PitchAngle_[rad]) -> MuxDynState/5(P [rad])  "PitchAngle_[rad]"
  Bicycle_model_[XYZ]/3(vz_[ms-1]) -> MuxDynState/3(vz [ms-1])  "Vz_[ms-1]"
  [YawRate] -> RearTyre/3(dpsi_[rads-1])
  [vy] -> RearTyre/2(vy_[ms-1])
  [Absvx] -> RearTyre/1(|vx|_[ms-1])
  [YawRate] -> FrontTyre/4(dYawAngle_[rads-1])
  [vy] -> FrontTyre/3(vy_[ms-1])
  [Absvx] -> FrontTyre/2(|vx|_[ms-1])
  [DeltaWheel] -> FrontTyre/1(DeltaWheel_[rad])
  Bicycle_model_[XYZ]/6(YawAngle_[rads-1]) -> [YawRate]  "YawRate_[rad s-1]"
  Bicycle_model_[XYZ]/4(RollAngle_[rad]) -> [RollAngle], MuxDynState/4(R [rad])  "RollAngle_[rad]"
  Bicycle_model_[XYZ]/2(vy_[ms-1]) -> MuxDynState/2(vy [ms-1]), [vy]  "Vy_[ms-1]"
  Bicycle_model_[XYZ]/1(|vx|_[ms-1]1) -> [Absvx]  "|vx|_[ms-1]"
  FrontTyre/1(FyFront_[N]) -> Bicycle_model_[XYZ]/6(Fy_front_[N])  "Fy_front_[N]"
  RearTyre/1(FyRear_[N]) -> Bicycle_model_[XYZ]/5(Fy_rear_[N])  "Fy_rear_[N]"
  SteerRatio/1 -> Bicycle_model_[XYZ]/1(DeltaWheel_[rad]), [DeltaWheel]  "DeltaWheel_[rad]"
  [vx] -> Abs/1
  Degrees to Radians/1 -> SteerRatio/1
  Abs/1 -> Bicycle_model_[XYZ]/4(|vx|_[ms-1])
  Bicycle_model_[XYZ]/9(ay_[ms-2]) -> ay_[ms-2]/1  "ay_[ms-2]"
  [DT] -> Product/2
  Product/1 -> to_kW/1
  Gain/1 -> Product/1
  to_kW/1 -> PDrive_[kW]/1  "PDrive_[kW]"
  [vy] -> Vy_[ms-1]/1  "vy_[ms-1]"

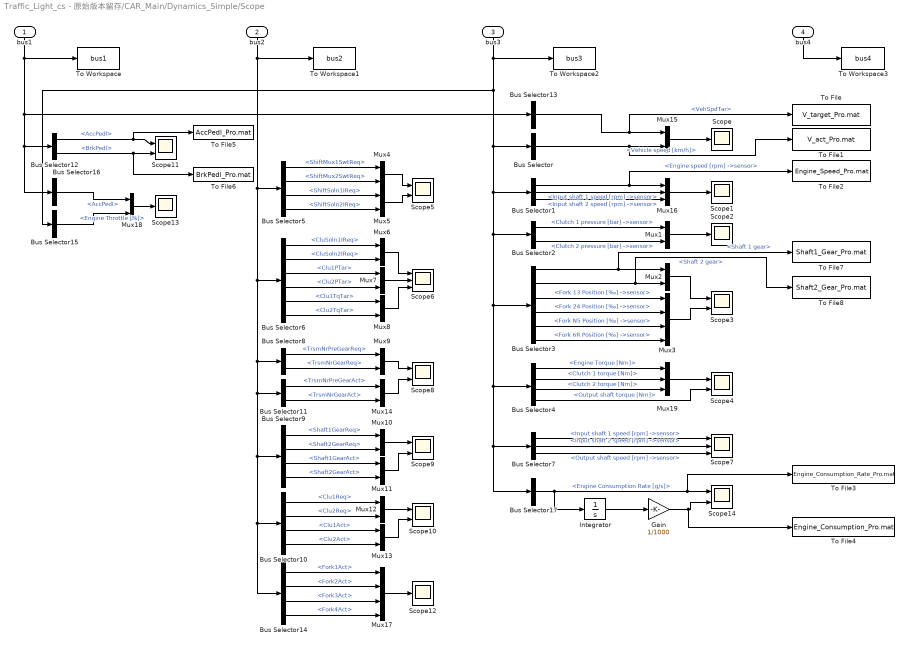
== system Traffic_Light_cs - 原始版本留存/CAR_Main/Dynamics_Simple/Scope ==
  bus1 : Inport
  bus2 : Inport  Port=2
  bus3 : Inport  Port=3
  bus4 : Inport  Port=4
  Bus Selector : BusSelector  OutputSignals=Vehicle speed [km/h]
  Bus Selector1 : BusSelector  OutputSignals=Engine speed [rpm] ->sensor,Input shaft 1 speed [rpm] ->sensor,Input shaft 2 speed [rpm] ->sensor
  Bus Selector10 : BusSelector  OutputSignals=Clu1Req,Clu2Req,Clu1Act,Clu2Act
  Bus Selector11 : BusSelector  OutputSignals=TrsmNrPreGearAct,TrsmNrGearAct
  Bus Selector12 : BusSelector  OutputSignals=AccPedl,BrkPedl
  Bus Selector13 : BusSelector  OutputSignals=VehSpdTar
  Bus Selector14 : BusSelector  OutputSignals=Fork1Act,Fork2Act,Fork3Act,Fork4Act
  Bus Selector15 : BusSelector  OutputSignals=Engine Throttle [%]
  Bus Selector16 : BusSelector  OutputSignals=AccPedl
  Bus Selector17 : BusSelector  OutputSignals=Engine Consumption Rate [g/s]
  Bus Selector2 : BusSelector  OutputSignals=Clutch 1 pressure [bar] ->sensor,Clutch 2 pressure [bar] ->sensor
  Bus Selector3 : BusSelector  OutputSignals=Shaft 1 gear,Shaft 2 gear,Fork 13 Position [‰] ->sensor,Fork 24 Position [‰] ->sensor,Fork N5 Position [‰] ->sensor,Fork 6R Position [‰] ->sensor
  Bus Selector4 : BusSelector  OutputSignals=Engine Torque [Nm],Clutch 1 torque [Nm],Clutch 2 torque [Nm],Output shaft torque [Nm]
  Bus Selector5 : BusSelector  OutputSignals=ShiftMux1SwtReq,ShiftMux2SwtReq,ShiftSoln1IReq,ShiftSoln2IReq
  Bus Selector6 : BusSelector  OutputSignals=CluSoln1IReq,CluSoln2IReq,Clu1PTar,Clu2PTar,Clu1TqTar,Clu2TqTar
  Bus Selector7 : BusSelector  OutputSignals=Input shaft 1 speed [rpm] ->sensor,Input shaft 2 speed [rpm] ->sensor,Output shaft speed [rpm] ->sensor
  Bus Selector8 : BusSelector  OutputSignals=TrsmNrPreGearReq,TrsmNrGearReq
  Bus Selector9 : BusSelector  OutputSignals=Shaft1GearReq,Shaft2GearReq,Shaft1GearAct,Shaft2GearAct
  Gain : Gain  Gain=1/1000
  Integrator : Integrator
  Mux{1..2,4..15,18} (15 alike) : Mux  Inputs=2
  Mux16 : Mux  Inputs=3
  Mux17 : Mux
  Mux19 : Mux  Inputs=3
  Mux3 : Mux
  Scope{,1..2,12..13} (5 alike) : Scope
  Scope{3..5,8..11,14} (8 alike) : Scope  NumInputPorts=2
  Scope6 : Scope  NumInputPorts=3
  Scope7 : Scope  NumInputPorts=3
  To File : ToFile  Filename=V_target_Pro.mat  MatrixName=V_target
  To File1 : ToFile  Filename=V_act_Pro.mat  MatrixName=V_act
  To File2 : ToFile  Filename=Engine_Speed_Pro.mat  MatrixName=Engine_Speed
  To File3 : ToFile  Filename=Engine_Consumption_Rate_Pro.mat  MatrixName=Engine_Consumption_Rate
  To File4 : ToFile  Filename=Engine_Consumption_Pro.mat  MatrixName=Engine_Consumption
  To File5 : ToFile  Filename=AccPedl_Pro.mat  MatrixName=AccPedl
  To File6 : ToFile  Filename=BrkPedl_Pro.mat  MatrixName=BrkPedl
  To File7 : ToFile  Filename=Shaft1_Gear_Pro.mat  MatrixName=Shaft1_Gear
  To File8 : ToFile  Filename=Shaft2_Gear_Pro.mat  MatrixName=Shaft2_Gear
  To Workspace : ToWorkspace  VariableName=bus1  SaveFormat=Timeseries  SampleTime=-1
  To Workspace1 : ToWorkspace  VariableName=bus2  SaveFormat=Timeseries  SampleTime=-1
  To Workspace2 : ToWorkspace  VariableName=bus3  SaveFormat=Timeseries  SampleTime=-1
  To Workspace3 : ToWorkspace  VariableName=bus4  SaveFormat=Timeseries  SampleTime=-1
  wires:
  Bus Selector1/2 -> Mux16/2  "<Input shaft 1 speed [rpm] ->sensor>"
  Bus Selector1/1 -> Mux16/1, To File2/1  "<Engine speed [rpm] ->sensor>"
  Bus Selector1/3 -> Mux16/3  "<Input shaft 2 speed [rpm] ->sensor>"
  Bus Selector/1 -> Mux15/2, To File1/1  "<Vehicle speed [km/h]>"
  Mux1/1 -> Scope2/1
  Bus Selector2/1 -> Mux1/1  "<Clutch 1 pressure [bar] ->sensor>"
  Bus Selector2/2 -> Mux1/2  "<Clutch 2 pressure [bar] ->sensor>"
  Mux2/1 -> Scope3/1
  Bus Selector3/1 -> Mux2/1, To File7/1  "<Shaft 1 gear>"
  Bus Selector3/2 -> Mux2/2, To File8/1  "<Shaft 2 gear>"
  Bus Selector3/3 -> Mux3/1  "<Fork 13 Position [‰] ->sensor>"
  Bus Selector3/4 -> Mux3/2  "<Fork 24 Position [‰] ->sensor>"
  Bus Selector3/5 -> Mux3/3  "<Fork N5 Position [‰] ->sensor>"
  Bus Selector3/6 -> Mux3/4  "<Fork 6R Position [‰] ->sensor>"
  Mux3/1 -> Scope3/2
  Bus Selector4/3 -> Mux19/3  "<Clutch 2 torque [Nm]>"
  Bus Selector4/2 -> Mux19/2  "<Clutch 1 torque [Nm]>"
  Bus Selector4/1 -> Mux19/1  "<Engine Torque [Nm]>"
  Bus Selector5/1 -> Mux4/1  "<ShiftMux1SwtReq>"
  Bus Selector5/2 -> Mux4/2  "<ShiftMux2SwtReq>"
  Bus Selector5/3 -> Mux5/1  "<ShiftSoln1IReq>"
  Bus Selector5/4 -> Mux5/2  "<ShiftSoln2IReq>"
  Mux4/1 -> Scope5/1
  Mux5/1 -> Scope5/2
  Mux6/1 -> Scope6/1
  Bus Selector6/1 -> Mux6/1  "<CluSoln1IReq>"
  Bus Selector6/2 -> Mux6/2  "<CluSoln2IReq>"
  Bus Selector6/3 -> Mux7/1  "<Clu1PTar>"
  Bus Selector6/4 -> Mux7/2  "<Clu2PTar>"
  Bus Selector6/5 -> Mux8/1  "<Clu1TqTar>"
  Bus Selector6/6 -> Mux8/2  "<Clu2TqTar>"
  Mux7/1 -> Scope6/2
  Mux8/1 -> Scope6/3
  Bus Selector7/3 -> Scope7/3  "<Output shaft speed [rpm] ->sensor>"
  Bus Selector7/2 -> Scope7/2  "<Input shaft 2 speed [rpm] ->sensor>"
  Bus Selector7/1 -> Scope7/1  "<Input shaft 1 speed [rpm] ->sensor>"
  Mux9/1 -> Scope8/1
  Bus Selector8/1 -> Mux9/1  "<TrsmNrPreGearReq>"
  Bus Selector8/2 -> Mux9/2  "<TrsmNrGearReq>"
  Mux10/1 -> Scope9/1
  Bus Selector9/1 -> Mux10/1  "<Shaft1GearReq>"
  Bus Selector9/2 -> Mux10/2  "<Shaft2GearReq>"
  Bus Selector9/4 -> Mux11/2  "<Shaft2GearAct>"
  Bus Selector9/3 -> Mux11/1  "<Shaft1GearAct>"
  Mux11/1 -> Scope9/2
  Bus Selector10/2 -> Mux12/2  "<Clu2Req>"
  Bus Selector10/4 -> Mux13/2  "<Clu2Act>"
  Bus Selector10/3 -> Mux13/1  "<Clu1Act>"
  Bus Selector10/1 -> Mux12/1  "<Clu1Req>"
  Mux12/1 -> Scope10/1
  Mux13/1 -> Scope10/2
  Mux14/1 -> Scope8/2
  Bus Selector11/1 -> Mux14/1  "<TrsmNrPreGearAct>"
  Bus Selector11/2 -> Mux14/2  "<TrsmNrGearAct>"
  bus1/1 -> To Workspace/1, Bus Selector13/1, Bus Selector16/1, Bus Selector12/1
  Bus Selector12/1 -> Scope11/1, To File5/1  "<AccPedl>"
  Bus Selector12/2 -> Scope11/2, To File6/1  "<BrkPedl>"
  Bus Selector13/1 -> Mux15/1, To File/1  "<VehSpdTar>"
  Mux15/1 -> Scope/1
  Mux16/1 -> Scope1/1
  Bus Selector14/2 -> Mux17/2  "<Fork2Act>"
  Bus Selector14/4 -> Mux17/4  "<Fork4Act>"
  Bus Selector14/3 -> Mux17/3  "<Fork3Act>"
  Bus Selector14/1 -> Mux17/1  "<Fork1Act>"
  Mux17/1 -> Scope12/1
  bus2/1 -> To Workspace1/1, Bus Selector11/1, Bus Selector14/1, Bus Selector10/1, Bus Selector9/1, Bus Selector8/1, Bus Selector6/1, Bus Selector5/1
  Mux18/1 -> Scope13/1
  Bus Selector16/1 -> Mux18/1  "<AccPedl>"
  Bus Selector15/1 -> Mux18/2  "<Engine Throttle [%]>"
  bus3/1 -> To Workspace2/1, Bus Selector15/1, Bus Selector17/1, Bus Selector7/1, Bus Selector4/1, Bus Selector3/1, Bus Selector2/1, Bus Selector1/1, Bus Selector/1
  Mux19/1 -> Scope4/1
  Bus Selector4/4 -> Scope4/2  "<Output shaft torque [Nm]>"
  Bus Selector17/1 -> Integrator/1, Scope14/1, To File3/1  "<Engine Consumption Rate [g/s]>"
  Integrator/1 -> Gain/1
  Gain/1 -> Scope14/2, To File4/1
  bus4/1 -> To Workspace3/1

== system Traffic_Light_cs - 原始版本留存/CAR_Main/LaneMarkerSensor_1_Data/If Action Subsystem1 ==
  In1 : Inport
  In2 : Inport  Port=2
  Action Port : ActionPort  ActionPortLabel=if(u1 >= u2)
  Bus Selector : BusSelector  OutputSignals=DATA
  Selector : Selector  IndexOptions=Index vector (port)  Indices=[4]  OutputSizes=1
  Out1 : Outport
  wires:
  Bus Selector/1 -> Out1/1  "<DATA>"
  Selector/1 -> Bus Selector/1
  In1/1 -> Selector/1
  In2/1 -> Selector/2

== system Traffic_Light_cs - 原始版本留存/CAR_Main/LaneMarkerSensor_1_Data/If Action Subsystem2 ==
  In1 : Inport
  In2 : Inport  Port=2
  Action Port : ActionPort  ActionPortLabel=if(u1 >= u2)
  Bus Selector : BusSelector  OutputSignals=DATA
  Selector : Selector  IndexOptions=Index vector (port)  Indices=[4]  OutputSizes=1
  Out1 : Outport
  wires:
  Bus Selector/1 -> Out1/1  "<DATA>"
  Selector/1 -> Bus Selector/1
  In1/1 -> Selector/1
  In2/1 -> Selector/2

== system Traffic_Light_cs - 原始版本留存/CAR_Main/LaneMarkerSensor_1_Data/If Action Subsystem3 ==
  In1 : Inport
  In2 : Inport  Port=2
  Action Port : ActionPort  ActionPortLabel=if(u1 >= u2)
  Bus Selector : BusSelector  OutputSignals=DATA
  Selector : Selector  IndexOptions=Index vector (port)  Indices=[4]  OutputSizes=1
  Out1 : Outport
  wires:
  Bus Selector/1 -> Out1/1  "<DATA>"
  Selector/1 -> Bus Selector/1
  In1/1 -> Selector/1
  In2/1 -> Selector/2

== system Traffic_Light_cs - 原始版本留存/CAR_Main/LaneMarkerSensor_1_Data/If Action Subsystem4 ==
  In1 : Inport
  In2 : Inport  Port=2
  Action Port : ActionPort  ActionPortLabel=if(u1 >= u2)
  Bus Selector : BusSelector  OutputSignals=DATA
  Selector : Selector  IndexOptions=Index vector (port)  Indices=[4]  OutputSizes=1
  Out1 : Outport
  wires:
  Bus Selector/1 -> Out1/1  "<DATA>"
  Selector/1 -> Bus Selector/1
  In1/1 -> Selector/1
  In2/1 -> Selector/2

== system Traffic_Light_cs - 原始版本留存/CAR_Main/SELF_Demux/compas converter ==
  rotz [rad] : Inport
  cart2compas : Subsystem
  rad2deg : Gain  Gain=180/pi
  heading [deg] : Outport
  wires:
  rad2deg/1 -> cart2compas/1(Angle [deg])
  rotz [rad]/1 -> rad2deg/1
  cart2compas/1(heading [deg]) -> heading [deg]/1

== system Traffic_Light_cs - 原始版本留存/CAR_Main/Subsystem/Signal Builder ==
  Demux : Demux  Tag=STV Demux  Outputs=6
      settings: DisplayOption=none
  FromWs : FromWorkspace  Tag=STV FromWs  VariableName=tuvar
      SigBuilderData=|
      | common.afterFinalStr = 'Extrapolate'
      | common.sampleTime = 0
      | dataSet.timeRange = [0 200]
      | dataSet.name = 'Traffic Light GPS Information'
      | sbobj.Groups.Name = 'Traffic Light GPS Information'
      | sbobj.Groups.Signals(1).Name = 'ID==1,X'
      | sbobj.Groups.Signals(1).XData = [0 200]
      | sbobj.Groups.Signals(1).YData = [-610.5 -610.5]
      | sbobj.Groups.Signals(2).Name = 'ID==1,Y'
      | sbobj.Groups.Signals(2).XData = [0 200]
      | sbobj.Groups.Signals(2).YData = [362.27 362.27]
      | sbobj.Groups.Signals(3).Name = 'ID==2,X'
      | sbobj.Groups.Signals(3).XData = [0 200]
      | sbobj.Groups.Signals(3).YData = [-639.42 -639.42]
      | sbobj.Groups.Signals(4).Name = 'ID==2,Y'
      | sbobj.Groups.Signals(4).XData = [0 200]
      | sbobj.Groups.Signals(4).YData = [295.94 295.94]
      | sbobj.Groups.Signals(5).Name = 'ID==3,X'
      | sbobj.Groups.Signals(5).XData = [0 200]
      | sbobj.Groups.Signals(5).YData = [-718.98 -718.98]
      | sbobj.Groups.Signals(6).Name = 'ID==3,Y'
      | sbobj.Groups.Signals(6).XData = [0 200]
      | sbobj.Groups.Signals(6).YData = [201.74 201.74]
      | sbobj.Groups.TimeRange = [0 200]
  ID==1,X : Outport  Tag=STV Outport
  ID==1,Y : Outport  Tag=STV Outport  Port=2  VectorParamsAs1DForOutWhenUnconnected=off
  ID==2,X : Outport  Tag=STV Outport  Port=3  VectorParamsAs1DForOutWhenUnconnected=off
  ID==2,Y : Outport  Tag=STV Outport  Port=4  VectorParamsAs1DForOutWhenUnconnected=off
  ID==3,X : Outport  Tag=STV Outport  Port=5  VectorParamsAs1DForOutWhenUnconnected=off
  ID==3,Y : Outport  Tag=STV Outport  Port=6  VectorParamsAs1DForOutWhenUnconnected=off
  wires:
  Demux/6 -> ID==3,Y/1
  Demux/5 -> ID==3,X/1
  Demux/4 -> ID==2,Y/1
  Demux/3 -> ID==2,X/1
  Demux/2 -> ID==1,Y/1
  Demux/1 -> ID==1,X/1
  FromWs/1 -> Demux/1

== system Traffic_Light_cs - 原始版本留存/CAR_Main/Subsystem1/Subsystem ==
  note: 类型0代表黄灯，初设3s
      | 类型1代表红灯，初设62s
      | 类型2代表绿灯，初设56s
  light_time : Inport
  light_type : Inport  Port=2
  Add{,1..3} (4 alike) : Sum
  Constant : Constant  Value=0.001
  Constant1 : Constant  Value=90
  Constant2 : Constant  Value=28
  Constant3 : Constant  Value=2
  Constant4 : Constant  Value=0
  Constant5 : Constant  Value=0
  Multiport Switch : MultiPortSwitch  Inputs=4
  Out2 : Outport  VectorParamsAs1DForOutWhenUnconnected=off
  wires:
  Constant5/1 -> Multiport Switch/5
  Constant4/1 -> Multiport Switch/2
  Add/1 -> Multiport Switch/1
  Constant3/1 -> Add/2
  Add3/1 -> Multiport Switch/4
  light_time/1 -> Add2/1, Add3/1
  Constant2/1 -> Add3/2
  Add2/1 -> Multiport Switch/3
  Constant1/1 -> Add2/2
  Constant/1 -> Add1/2
  Add1/1 -> Out2/1
  Multiport Switch/1 -> Add1/1
  light_type/1 -> Add/1

== system Traffic_Light_cs - 原始版本留存/CAR_Ahead/Decision/Function-Call Subsystem/Subsystem ==
  Dis : Inport
  "CameraSensor " : Inport  Port=2
  function : TriggerPort  TriggerType=function-call  VariantControl=Variant
  CameraSensor_0919_100_CM_Demux : Subsystem  Tag=demux/Camera/Color  mask{SensorName=CameraSensor_0919_100, hres=1920, vres=1800}
      mask prompts: SensorName "Sensor Name"; hres "Horizontal Resolution"; vres "Vertical Resolution"
      mask Help: eval('openHelp(457)')
      mask Display:
      | fprintf('MONO CAMERA:\n Color\n %s \n %d x %d px',SensorName,hres,vres)
      | port_label('output',1,'R')
      | port_label('output',2,'G')
      | port_label('output',3,'B')
  Constant : Constant  Value=14
  Delay : Stateflow chart  TreatAsAtomicUnit=on
  MATLAB Function : MATLAB Function  TreatAsAtomicUnit=on
  Product : Product
  Sqrt : Sqrt  SaturateOnIntegerOverflow=on
  Sum : Sum  Inputs=|-+
  Light_State_Ahead : Outport  VectorParamsAs1DForOutWhenUnconnected=off
  wires:
  Delay/1(Light_State_End) -> Light_State_Ahead/1
  Sqrt/1 -> MATLAB Function/1(Dis)
  Sum/1 -> Sqrt/1
  Constant/1 -> Sum/1
  Product/1 -> Sum/2
  Dis/1 -> Product/2, Product/1
  [B_Ori] -> MATLAB Function/4(B_Ori)
  CameraSensor_0919_100_CM_Demux/3(B) -> [B_Ori]
  MATLAB Function/1(Light_State) -> Delay/1(Light_State_0919_100)  "Light_State_Ahead"
  CameraSensor_0919_100_CM_Demux/2(G) -> [G_Ori]
  CameraSensor_0919_100_CM_Demux/1(R) -> [R_Ori]
  "CameraSensor "/1 -> CameraSensor_0919_100_CM_Demux/1(In1)
  [G_Ori] -> MATLAB Function/3(G_Ori)
  [R_Ori] -> MATLAB Function/2(R_Ori)

== system Traffic_Light_cs - 原始版本留存/CAR_Ahead/SELF_Demux/compas converter/cart2compas ==
  Angle [deg] : Inport
  Constant : Constant  Value=90
  Constant1 : Constant  Value=360
  Gain : Gain  Gain=1/360
  Gain1 : Gain  Gain=360
  Gain2 : Gain  Gain=-1
  Rounding Function : Rounding
  Sum : Sum  Inputs=|-+
  Sum1 : Sum  Inputs=-+|
  Sum2 : Sum  Inputs=++|
  heading [deg] : Outport
  wires:
  Gain/1 -> Rounding Function/1
  Rounding Function/1 -> Gain1/1
  Gain1/1 -> Sum/1
  Angle [deg]/1 -> Sum1/2
  Sum/1 -> Gain2/1
  Sum1/1 -> Gain/1, Sum/2
  Constant/1 -> Sum1/1
  Gain2/1 -> Sum2/2
  Constant1/1 -> Sum2/1
  Sum2/1 -> heading [deg]/1

== system Traffic_Light_cs - 原始版本留存/CAR_Ahead/Trajectories/Traj2State1/Traj2State2 ==
  traj : Inport
  MuxState : Subsystem
  Traj2MuxState_Ext : Subsystem
  state : Outport
  wires:
  Traj2MuxState_Ext/9(Y [rad]) -> MuxState/9(Y [rad])
  Traj2MuxState_Ext/8(P [rad]) -> MuxState/8(P [rad])
  Traj2MuxState_Ext/7(R [rad]) -> MuxState/7(R [rad])
  Traj2MuxState_Ext/6(dz [m/s]) -> MuxState/6(dz [m/s])
  Traj2MuxState_Ext/5(dy [m/s]) -> MuxState/5(dy [m/s])
  Traj2MuxState_Ext/4(dx [m/s]) -> MuxState/4(dx [m/s])
  Traj2MuxState_Ext/3(z [m]) -> MuxState/3(z [m])
  Traj2MuxState_Ext/2(y [m]) -> MuxState/2(y [m])
  Traj2MuxState_Ext/1(x [m]) -> MuxState/1(x [m])
  MuxState/1(state) -> state/1
  traj/1 -> Traj2MuxState_Ext/1(Traj)
